simulink model "VCU_CS75_10_9_SteeringTorque"  (R2014a)
settings: Solver=FixedStepDiscrete  StartTime=0.0  StopTime=25  FixedStep=0.0005  RelTol=1e-3
undefined symbols (not defined in the file or in its folder): AutoDrivingReady, ecucoder_acal, I_SW01_L, LaterlAngleCommand, LDW, RemoteAcclPosition
libraries: simulink x880, ec5744lib x37
(part 14 of 30)

== system VCU_CS75_10_9_SteeringTorque/长安CS75底盘程序，20ms一次/Output/CAN0_Tx/to6001/A/Wheel_Speed_RR_Data ==
  Wheel_Speed_RR_Data : Inport
  Constant{1..6} (6 alike) : Constant  Value=0  OutDataTypeStr=uint8
  Wheel_Speed_RR_DataABS : Abs
  Wheel_Speed_RR_DataBitCov : DataTypeConversion  OutDataTypeStr=uint8
  Wheel_Speed_RR_DataCOV : DataTypeConversion  OutDataTypeStr=uint8
  Wheel_Speed_RR_DataCS : ArithShift  BitShiftNumber=-16
  Wheel_Speed_RR_DataConS : Constant  OutDataTypeStr=single
  Wheel_Speed_RR_DataCosR : Constant  Value=0  OutDataTypeStr=uint8
  Wheel_Speed_RR_DataROP : RelationalOperator  Operator=<  OutDataTypeStr=boolean
  Wheel_Speed_RR_DataRon : Rounding  Operator=round
  Wheel_Speed_RR_DataSW : Switch  Criteria=u2 ~= 0
  Wheel_Speed_RR_Data_1sat : Saturate  UpperLimit=65535  LowerLimit=0
  Wheel_Speed_RR_Data_And : simulink/Logic and Bit Operations/Bitwise Operator  logicop=AND  UseBitMask=off  NumInputPorts=2  BitMask=bin2dec('11011001')  BitMaskRealWorld=Stored Integer
  Wheel_Speed_RR_Data_And_C : Constant  Value=255  OutDataTypeStr=uint32
  Wheel_Speed_RR_Data_Convert : DataTypeConversion  OutDataTypeStr=uint32
  Wheel_Speed_RR_Data_D : Product  Inputs=*/
  Wheel_Speed_RR_Data_D1 : Product  Inputs=*/
  Wheel_Speed_RR_Data_F : Constant  Value=0.05625  OutDataTypeStr=single
  Wheel_Speed_RR_Data_L : simulink/Logic and Bit Operations/Bitwise Operator  logicop=AND  UseBitMask=on  BitMask=65535  BitMaskRealWorld=Stored Integer
  Wheel_Speed_RR_Data_O : Constant  Value=0  OutDataTypeStr=single
  Wheel_Speed_RR_Data_S : ArithShift
  Wheel_Speed_RR_Data_sat : Saturate  UpperLimit=200  LowerLimit=-200
  Wheel_Speed_RR_Data_st : Sum  Inputs=+-
  Wheel_Speed_RR_Dataoutput7_C : Constant  Value=256
  Wheel_Speed_RR_Datasubcon : Sum  Inputs=+-
  output1 : Outport
  output2 : Outport  Port=2
  output3 : Outport  Port=3
  output4 : Outport  Port=4
  output5 : Outport  Port=5
  output6 : Outport  Port=6
  output7 : Outport  Port=7
  output8 : Outport  Port=8
  wires:
  Constant6/1 -> output6/1
  Constant5/1 -> output5/1
  Constant4/1 -> output4/1
  Constant3/1 -> output3/1
  Constant2/1 -> output2/1
  Constant1/1 -> output1/1
  Wheel_Speed_RR_DataBitCov/1 -> output8/1
  Wheel_Speed_RR_Data_And/1 -> Wheel_Speed_RR_DataBitCov/1
  Wheel_Speed_RR_Data_And_C/1 -> Wheel_Speed_RR_Data_And/2
  Wheel_Speed_RR_DataCOV/1 -> output7/1
  Wheel_Speed_RR_Data_D1/1 -> Wheel_Speed_RR_DataCOV/1
  Wheel_Speed_RR_Dataoutput7_C/1 -> Wheel_Speed_RR_Data_D1/2
  Wheel_Speed_RR_Data_L/1 -> Wheel_Speed_RR_Data_And/1, Wheel_Speed_RR_Data_D1/1
  Wheel_Speed_RR_Data_Convert/1 -> Wheel_Speed_RR_Data_L/1
  Wheel_Speed_RR_Data_1sat/1 -> Wheel_Speed_RR_Data_Convert/1
  Wheel_Speed_RR_Data_S/1 -> Wheel_Speed_RR_Data_1sat/1
  Wheel_Speed_RR_DataSW/1 -> Wheel_Speed_RR_Data_S/1
  Wheel_Speed_RR_DataROP/1 -> Wheel_Speed_RR_DataSW/2
  Wheel_Speed_RR_Datasubcon/1 -> Wheel_Speed_RR_DataSW/1
  Wheel_Speed_RR_DataABS/1 -> Wheel_Speed_RR_Datasubcon/2
  Wheel_Speed_RR_DataCS/1 -> Wheel_Speed_RR_Datasubcon/1
  Wheel_Speed_RR_DataConS/1 -> Wheel_Speed_RR_DataCS/1
  Wheel_Speed_RR_DataCosR/1 -> Wheel_Speed_RR_DataROP/2
  Wheel_Speed_RR_DataRon/1 -> Wheel_Speed_RR_DataSW/3, Wheel_Speed_RR_DataABS/1, Wheel_Speed_RR_DataROP/1
  Wheel_Speed_RR_Data_D/1 -> Wheel_Speed_RR_DataRon/1
  Wheel_Speed_RR_Data_F/1 -> Wheel_Speed_RR_Data_D/2
  Wheel_Speed_RR_Data_st/1 -> Wheel_Speed_RR_Data_D/1
  Wheel_Speed_RR_Data_O/1 -> Wheel_Speed_RR_Data_st/2
  Wheel_Speed_RR_Data_sat/1 -> Wheel_Speed_RR_Data_st/1
  Wheel_Speed_RR_Data/1 -> Wheel_Speed_RR_Data_sat/1

== system VCU_CS75_10_9_SteeringTorque/长安CS75底盘程序，20ms一次/Output/CAN0_Tx/to6002/B/BrakePeadlState ==
  BrakePeadlState : Inport
  BrakePeadlStateRon : Rounding  Operator=round
  BrakePeadlState_1sat : Saturate  UpperLimit=255  LowerLimit=0
  BrakePeadlState_Convert : DataTypeConversion  OutDataTypeStr=uint8
  BrakePeadlState_Convert1 : DataTypeConversion  OutDataTypeStr=uint32
  BrakePeadlState_D : Product  Inputs=*/
  BrakePeadlState_F : Constant  OutDataTypeStr=single
  BrakePeadlState_L : simulink/Logic and Bit Operations/Bitwise Operator  logicop=AND  UseBitMask=on  BitMask=255  BitMaskRealWorld=Stored Integer
  BrakePeadlState_O : Constant  Value=0  OutDataTypeStr=single
  BrakePeadlState_S : ArithShift
  BrakePeadlState_sat : Saturate  UpperLimit=3  LowerLimit=0
  BrakePeadlState_st : Sum  Inputs=+-
  Constant{1..5,7..8} (7 alike) : Constant  Value=0  OutDataTypeStr=uint8
  output1 : Outport
  output2 : Outport  Port=2
  output3 : Outport  Port=3
  output4 : Outport  Port=4
  output5 : Outport  Port=5
  output6 : Outport  Port=6
  output7 : Outport  Port=7
  output8 : Outport  Port=8
  wires:
  BrakePeadlState/1 -> BrakePeadlState_sat/1
  BrakePeadlState_sat/1 -> BrakePeadlState_st/1
  BrakePeadlState_O/1 -> BrakePeadlState_st/2
  BrakePeadlState_st/1 -> BrakePeadlState_D/1
  BrakePeadlState_F/1 -> BrakePeadlState_D/2
  BrakePeadlState_D/1 -> BrakePeadlStateRon/1
  BrakePeadlStateRon/1 -> BrakePeadlState_S/1
  BrakePeadlState_S/1 -> BrakePeadlState_1sat/1
  BrakePeadlState_1sat/1 -> BrakePeadlState_Convert1/1
  BrakePeadlState_Convert1/1 -> BrakePeadlState_L/1
  BrakePeadlState_L/1 -> BrakePeadlState_Convert/1
  BrakePeadlState_Convert/1 -> output6/1
  Constant1/1 -> output1/1
  Constant2/1 -> output2/1
  Constant3/1 -> output3/1
  Constant4/1 -> output4/1
  Constant5/1 -> output5/1
  Constant7/1 -> output7/1
  Constant8/1 -> output8/1

== system VCU_CS75_10_9_SteeringTorque/长安CS75底盘程序，20ms一次/Output/CAN0_Tx/to6002/B/RemoteDecelerationRequest ==
  RemoteDecelerationRequest : Inport
  Constant{1..7} (7 alike) : Constant  Value=0  OutDataTypeStr=uint8
  RemoteDecelerationRequestRon : Rounding  Operator=round
  RemoteDecelerationRequest_1sat : Saturate  UpperLimit=255  LowerLimit=0
  RemoteDecelerationRequest_Convert : DataTypeConversion  OutDataTypeStr=uint8
  RemoteDecelerationRequest_Convert1 : DataTypeConversion  OutDataTypeStr=uint32
  RemoteDecelerationRequest_D : Product  Inputs=*/
  RemoteDecelerationRequest_F : Constant  Value=0.05  OutDataTypeStr=single
  RemoteDecelerationRequest_L : simulink/Logic and Bit Operations/Bitwise Operator  logicop=AND  UseBitMask=on  BitMask=255  BitMaskRealWorld=Stored Integer
  RemoteDecelerationRequest_O : Constant  Value=0  OutDataTypeStr=single
  RemoteDecelerationRequest_S : ArithShift
  RemoteDecelerationRequest_sat : Saturate  UpperLimit=12.75  LowerLimit=0
  RemoteDecelerationRequest_st : Sum  Inputs=+-
  output1 : Outport
  output2 : Outport  Port=2
  output3 : Outport  Port=3
  output4 : Outport  Port=4
  output5 : Outport  Port=5
  output6 : Outport  Port=6
  output7 : Outport  Port=7
  output8 : Outport  Port=8
  wires:
  RemoteDecelerationRequest/1 -> RemoteDecelerationRequest_sat/1
  RemoteDecelerationRequest_sat/1 -> RemoteDecelerationRequest_st/1
  RemoteDecelerationRequest_O/1 -> RemoteDecelerationRequest_st/2
  RemoteDecelerationRequest_st/1 -> RemoteDecelerationRequest_D/1
  RemoteDecelerationRequest_F/1 -> RemoteDecelerationRequest_D/2
  RemoteDecelerationRequest_D/1 -> RemoteDecelerationRequestRon/1
  RemoteDecelerationRequestRon/1 -> RemoteDecelerationRequest_S/1
  RemoteDecelerationRequest_S/1 -> RemoteDecelerationRequest_1sat/1
  RemoteDecelerationRequest_1sat/1 -> RemoteDecelerationRequest_Convert1/1
  RemoteDecelerationRequest_Convert1/1 -> RemoteDecelerationRequest_L/1
  RemoteDecelerationRequest_L/1 -> RemoteDecelerationRequest_Convert/1
  RemoteDecelerationRequest_Convert/1 -> output8/1
  Constant1/1 -> output1/1
  Constant2/1 -> output2/1
  Constant3/1 -> output3/1
  Constant4/1 -> output4/1
  Constant5/1 -> output5/1
  Constant6/1 -> output6/1
  Constant7/1 -> output7/1

== system VCU_CS75_10_9_SteeringTorque/长安CS75底盘程序，20ms一次/Output/CAN0_Tx/to6002/B/RemoteThrottlePercentage ==
  RemoteThrottlePercentage : Inport
  Constant{1..6,8} (7 alike) : Constant  Value=0  OutDataTypeStr=uint8
  RemoteThrottlePercentageRon : Rounding  Operator=round
  RemoteThrottlePercentage_1sat : Saturate  UpperLimit=255  LowerLimit=0
  RemoteThrottlePercentage_Convert : DataTypeConversion  OutDataTypeStr=uint8
  RemoteThrottlePercentage_Convert1 : DataTypeConversion  OutDataTypeStr=uint32
  RemoteThrottlePercentage_D : Product  Inputs=*/
  RemoteThrottlePercentage_F : Constant  Value=0.4  OutDataTypeStr=single
  RemoteThrottlePercentage_L : simulink/Logic and Bit Operations/Bitwise Operator  logicop=AND  UseBitMask=on  BitMask=255  BitMaskRealWorld=Stored Integer
  RemoteThrottlePercentage_O : Constant  Value=0  OutDataTypeStr=single
  RemoteThrottlePercentage_S : ArithShift
  RemoteThrottlePercentage_sat : Saturate  UpperLimit=100  LowerLimit=0
  RemoteThrottlePercentage_st : Sum  Inputs=+-
  output1 : Outport
  output2 : Outport  Port=2
  output3 : Outport  Port=3
  output4 : Outport  Port=4
  output5 : Outport  Port=5
  output6 : Outport  Port=6
  output7 : Outport  Port=7
  output8 : Outport  Port=8
  wires:
  RemoteThrottlePercentage/1 -> RemoteThrottlePercentage_sat/1
  RemoteThrottlePercentage_sat/1 -> RemoteThrottlePercentage_st/1
  RemoteThrottlePercentage_O/1 -> RemoteThrottlePercentage_st/2
  RemoteThrottlePercentage_st/1 -> RemoteThrottlePercentage_D/1
  RemoteThrottlePercentage_F/1 -> RemoteThrottlePercentage_D/2
  RemoteThrottlePercentage_D/1 -> RemoteThrottlePercentageRon/1
  RemoteThrottlePercentageRon/1 -> RemoteThrottlePercentage_S/1
  RemoteThrottlePercentage_S/1 -> RemoteThrottlePercentage_1sat/1
  RemoteThrottlePercentage_1sat/1 -> RemoteThrottlePercentage_Convert1/1
  RemoteThrottlePercentage_Convert1/1 -> RemoteThrottlePercentage_L/1
  RemoteThrottlePercentage_L/1 -> RemoteThrottlePercentage_Convert/1
  RemoteThrottlePercentage_Convert/1 -> output7/1
  Constant1/1 -> output1/1
  Constant2/1 -> output2/1
  Constant3/1 -> output3/1
  Constant4/1 -> output4/1
  Constant5/1 -> output5/1
  Constant6/1 -> output6/1
  Constant8/1 -> output8/1

== system VCU_CS75_10_9_SteeringTorque/长安CS75底盘程序，20ms一次/Output/CAN0_Tx/to6002/B/Steering_Angle ==
  Steering_Angle : Inport
  Constant{1..2,5..8} (6 alike) : Constant  Value=0  OutDataTypeStr=uint8
  Steering_AngleABS : Abs
  Steering_AngleBitCov : DataTypeConversion  OutDataTypeStr=uint8
  Steering_AngleCOV : DataTypeConversion  OutDataTypeStr=uint8
  Steering_AngleCS : ArithShift  BitShiftNumber=-16
  Steering_AngleConS : Constant  OutDataTypeStr=single
  Steering_AngleCosR : Constant  Value=0  OutDataTypeStr=uint8
  Steering_AngleROP : RelationalOperator  Operator=<  OutDataTypeStr=boolean
  Steering_AngleRon : Rounding  Operator=round
  Steering_AngleSW : Switch  Criteria=u2 ~= 0
  Steering_Angle_1sat : Saturate  UpperLimit=65535  LowerLimit=0
  Steering_Angle_And : simulink/Logic and Bit Operations/Bitwise Operator  logicop=AND  UseBitMask=off  NumInputPorts=2  BitMask=bin2dec('11011001')  BitMaskRealWorld=Stored Integer
  Steering_Angle_And_C : Constant  Value=255  OutDataTypeStr=uint32
  Steering_Angle_Convert : DataTypeConversion  OutDataTypeStr=uint32
  Steering_Angle_D : Product  Inputs=*/
  Steering_Angle_D1 : Product  Inputs=*/
  Steering_Angle_F : Constant  Value=0.1  OutDataTypeStr=single
  Steering_Angle_L : simulink/Logic and Bit Operations/Bitwise Operator  logicop=AND  UseBitMask=on  BitMask=65535  BitMaskRealWorld=Stored Integer
  Steering_Angle_O : Constant  Value=0  OutDataTypeStr=single
  Steering_Angle_S : ArithShift
  Steering_Angle_sat : Saturate  UpperLimit=780  LowerLimit=-780
  Steering_Angle_st : Sum  Inputs=+-
  Steering_Angleoutput3_C : Constant  Value=256
  Steering_Anglesubcon : Sum  Inputs=+-
  output1 : Outport
  output2 : Outport  Port=2
  output3 : Outport  Port=3
  output4 : Outport  Port=4
  output5 : Outport  Port=5
  output6 : Outport  Port=6
  output7 : Outport  Port=7
  output8 : Outport  Port=8
  wires:
  Steering_Angle/1 -> Steering_Angle_sat/1
  Steering_Angle_sat/1 -> Steering_Angle_st/1
  Steering_Angle_O/1 -> Steering_Angle_st/2
  Steering_Angle_st/1 -> Steering_Angle_D/1
  Steering_Angle_F/1 -> Steering_Angle_D/2
  Steering_Angle_D/1 -> Steering_AngleRon/1
  Steering_AngleRon/1 -> Steering_AngleROP/1, Steering_AngleABS/1, Steering_AngleSW/3
  Steering_AngleCosR/1 -> Steering_AngleROP/2
  Steering_AngleConS/1 -> Steering_AngleCS/1
  Steering_AngleCS/1 -> Steering_Anglesubcon/1
  Steering_AngleABS/1 -> Steering_Anglesubcon/2
  Steering_Anglesubcon/1 -> Steering_AngleSW/1
  Steering_AngleROP/1 -> Steering_AngleSW/2
  Steering_AngleSW/1 -> Steering_Angle_S/1
  Steering_Angle_S/1 -> Steering_Angle_1sat/1
  Steering_Angle_1sat/1 -> Steering_Angle_Convert/1
  Steering_Angle_Convert/1 -> Steering_Angle_L/1
  Steering_Angle_L/1 -> Steering_Angle_D1/1, Steering_Angle_And/1
  Steering_Angleoutput3_C/1 -> Steering_Angle_D1/2
  Steering_Angle_D1/1 -> Steering_AngleCOV/1
  Steering_AngleCOV/1 -> output3/1
  Steering_Angle_And_C/1 -> Steering_Angle_And/2
  Steering_Angle_And/1 -> Steering_AngleBitCov/1
  Steering_AngleBitCov/1 -> output4/1
  Constant1/1 -> output1/1
  Constant2/1 -> output2/1
  Constant5/1 -> output5/1
  Constant6/1 -> output6/1
  Constant7/1 -> output7/1
  Constant8/1 -> output8/1

== system VCU_CS75_10_9_SteeringTorque/长安CS75底盘程序，20ms一次/Output/CAN0_Tx/to6002/B/ThrottlePedalPercentage ==
  ThrottlePedalPercentage : Inport
  Constant{1..4,6..8} (7 alike) : Constant  Value=0  OutDataTypeStr=uint8
  ThrottlePedalPercentageRon : Rounding  Operator=round
  ThrottlePedalPercentage_1sat : Saturate  UpperLimit=255  LowerLimit=0
  ThrottlePedalPercentage_Convert : DataTypeConversion  OutDataTypeStr=uint8
  ThrottlePedalPercentage_Convert1 : DataTypeConversion  OutDataTypeStr=uint32
  ThrottlePedalPercentage_D : Product  Inputs=*/
  ThrottlePedalPercentage_F : Constant  Value=0.4  OutDataTypeStr=single
  ThrottlePedalPercentage_L : simulink/Logic and Bit Operations/Bitwise Operator  logicop=AND  UseBitMask=on  BitMask=255  BitMaskRealWorld=Stored Integer
  ThrottlePedalPercentage_O : Constant  Value=0  OutDataTypeStr=single
  ThrottlePedalPercentage_S : ArithShift
  ThrottlePedalPercentage_sat : Saturate  UpperLimit=100  LowerLimit=0
  ThrottlePedalPercentage_st : Sum  Inputs=+-
  output1 : Outport
  output2 : Outport  Port=2
  output3 : Outport  Port=3
  output4 : Outport  Port=4
  output5 : Outport  Port=5
  output6 : Outport  Port=6
  output7 : Outport  Port=7
  output8 : Outport  Port=8
  wires:
  ThrottlePedalPercentage/1 -> ThrottlePedalPercentage_sat/1
  ThrottlePedalPercentage_sat/1 -> ThrottlePedalPercentage_st/1
  ThrottlePedalPercentage_O/1 -> ThrottlePedalPercentage_st/2
  ThrottlePedalPercentage_st/1 -> ThrottlePedalPercentage_D/1
  ThrottlePedalPercentage_F/1 -> ThrottlePedalPercentage_D/2
  ThrottlePedalPercentage_D/1 -> ThrottlePedalPercentageRon/1
  ThrottlePedalPercentageRon/1 -> ThrottlePedalPercentage_S/1
  ThrottlePedalPercentage_S/1 -> ThrottlePedalPercentage_1sat/1
  ThrottlePedalPercentage_1sat/1 -> ThrottlePedalPercentage_Convert1/1
  ThrottlePedalPercentage_Convert1/1 -> ThrottlePedalPercentage_L/1
  ThrottlePedalPercentage_L/1 -> ThrottlePedalPercentage_Convert/1
  ThrottlePedalPercentage_Convert/1 -> output5/1
  Constant1/1 -> output1/1
  Constant2/1 -> output2/1
  Constant3/1 -> output3/1
  Constant4/1 -> output4/1
  Constant6/1 -> output6/1
  Constant7/1 -> output7/1
  Constant8/1 -> output8/1

== system VCU_CS75_10_9_SteeringTorque/长安CS75底盘程序，20ms一次/Output/CAN0_Tx/to6002/B/VehicleSpeed ==
  VehicleSpeed : Inport
  Constant{3..8} (6 alike) : Constant  Value=0  OutDataTypeStr=uint8
  VehicleSpeedABS : Abs
  VehicleSpeedBitCov : DataTypeConversion  OutDataTypeStr=uint8
  VehicleSpeedCOV : DataTypeConversion  OutDataTypeStr=uint8
  VehicleSpeedCS : ArithShift  BitShiftNumber=-16
  VehicleSpeedConS : Constant  OutDataTypeStr=single
  VehicleSpeedCosR : Constant  Value=0  OutDataTypeStr=uint8
  VehicleSpeedROP : RelationalOperator  Operator=<  OutDataTypeStr=boolean
  VehicleSpeedRon : Rounding  Operator=round
  VehicleSpeedSW : Switch  Criteria=u2 ~= 0
  VehicleSpeed_1sat : Saturate  UpperLimit=65535  LowerLimit=0
  VehicleSpeed_And : simulink/Logic and Bit Operations/Bitwise Operator  logicop=AND  UseBitMask=off  NumInputPorts=2  BitMask=bin2dec('11011001')  BitMaskRealWorld=Stored Integer
  VehicleSpeed_And_C : Constant  Value=255  OutDataTypeStr=uint32
  VehicleSpeed_Convert : DataTypeConversion  OutDataTypeStr=uint32
  VehicleSpeed_D : Product  Inputs=*/
  VehicleSpeed_D1 : Product  Inputs=*/
  VehicleSpeed_F : Constant  Value=0.05625  OutDataTypeStr=single
  VehicleSpeed_L : simulink/Logic and Bit Operations/Bitwise Operator  logicop=AND  UseBitMask=on  BitMask=65535  BitMaskRealWorld=Stored Integer
  VehicleSpeed_O : Constant  Value=0  OutDataTypeStr=single
  VehicleSpeed_S : ArithShift
  VehicleSpeed_sat : Saturate  UpperLimit=200  LowerLimit=-200
  VehicleSpeed_st : Sum  Inputs=+-
  VehicleSpeedoutput1_C : Constant  Value=256
  VehicleSpeedsubcon : Sum  Inputs=+-
  output1 : Outport
  output2 : Outport  Port=2
  output3 : Outport  Port=3
  output4 : Outport  Port=4
  output5 : Outport  Port=5
  output6 : Outport  Port=6
  output7 : Outport  Port=7
  output8 : Outport  Port=8
  wires:
  VehicleSpeed/1 -> VehicleSpeed_sat/1
  VehicleSpeed_sat/1 -> VehicleSpeed_st/1
  VehicleSpeed_O/1 -> VehicleSpeed_st/2
  VehicleSpeed_st/1 -> VehicleSpeed_D/1
  VehicleSpeed_F/1 -> VehicleSpeed_D/2
  VehicleSpeed_D/1 -> VehicleSpeedRon/1
  VehicleSpeedRon/1 -> VehicleSpeedROP/1, VehicleSpeedABS/1, VehicleSpeedSW/3
  VehicleSpeedCosR/1 -> VehicleSpeedROP/2
  VehicleSpeedConS/1 -> VehicleSpeedCS/1
  VehicleSpeedCS/1 -> VehicleSpeedsubcon/1
  VehicleSpeedABS/1 -> VehicleSpeedsubcon/2
  VehicleSpeedsubcon/1 -> VehicleSpeedSW/1
  VehicleSpeedROP/1 -> VehicleSpeedSW/2
  VehicleSpeedSW/1 -> VehicleSpeed_S/1
  VehicleSpeed_S/1 -> VehicleSpeed_1sat/1
  VehicleSpeed_1sat/1 -> VehicleSpeed_Convert/1
  VehicleSpeed_Convert/1 -> VehicleSpeed_L/1
  VehicleSpeed_L/1 -> VehicleSpeed_D1/1, VehicleSpeed_And/1
  VehicleSpeedoutput1_C/1 -> VehicleSpeed_D1/2
  VehicleSpeed_D1/1 -> VehicleSpeedCOV/1
  VehicleSpeedCOV/1 -> output1/1
  VehicleSpeed_And_C/1 -> VehicleSpeed_And/2
  VehicleSpeed_And/1 -> VehicleSpeedBitCov/1
  VehicleSpeedBitCov/1 -> output2/1
  Constant3/1 -> output3/1
  Constant4/1 -> output4/1
  Constant5/1 -> output5/1
  Constant6/1 -> output6/1
  Constant7/1 -> output7/1
  Constant8/1 -> output8/1

== system VCU_CS75_10_9_SteeringTorque/长安CS75底盘程序，20ms一次/Output/CAN0_Tx/to6003/C/LateralAcceleration ==
  LateralAcceleration : Inport
  Constant{1..2,4..8} (7 alike) : Constant  Value=0  OutDataTypeStr=uint8
  LateralAccelerationRon : Rounding  Operator=round
  LateralAcceleration_1sat : Saturate  UpperLimit=255  LowerLimit=0
  LateralAcceleration_Convert : DataTypeConversion  OutDataTypeStr=uint8
  LateralAcceleration_Convert1 : DataTypeConversion  OutDataTypeStr=uint32
  LateralAcceleration_D : Product  Inputs=*/
  LateralAcceleration_F : Constant  Value=0.1  OutDataTypeStr=single
  LateralAcceleration_L : simulink/Logic and Bit Operations/Bitwise Operator  logicop=AND  UseBitMask=on  BitMask=255  BitMaskRealWorld=Stored Integer
  LateralAcceleration_O : Constant  Value=-12.7  OutDataTypeStr=single
  LateralAcceleration_S : ArithShift
  LateralAcceleration_sat : Saturate  UpperLimit=12.8  LowerLimit=-12.7
  LateralAcceleration_st : Sum  Inputs=+-
  output1 : Outport
  output2 : Outport  Port=2
  output3 : Outport  Port=3
  output4 : Outport  Port=4
  output5 : Outport  Port=5
  output6 : Outport  Port=6
  output7 : Outport  Port=7
  output8 : Outport  Port=8
  wires:
  LateralAcceleration/1 -> LateralAcceleration_sat/1
  LateralAcceleration_sat/1 -> LateralAcceleration_st/1
  LateralAcceleration_O/1 -> LateralAcceleration_st/2
  LateralAcceleration_st/1 -> LateralAcceleration_D/1
  LateralAcceleration_F/1 -> LateralAcceleration_D/2
  LateralAcceleration_D/1 -> LateralAccelerationRon/1
  LateralAccelerationRon/1 -> LateralAcceleration_S/1
  LateralAcceleration_S/1 -> LateralAcceleration_1sat/1
  LateralAcceleration_1sat/1 -> LateralAcceleration_Convert1/1
  LateralAcceleration_Convert1/1 -> LateralAcceleration_L/1
  LateralAcceleration_L/1 -> LateralAcceleration_Convert/1
  LateralAcceleration_Convert/1 -> output3/1
  Constant1/1 -> output1/1
  Constant2/1 -> output2/1
  Constant4/1 -> output4/1
  Constant5/1 -> output5/1
  Constant6/1 -> output6/1
  Constant7/1 -> output7/1
  Constant8/1 -> output8/1

== system VCU_CS75_10_9_SteeringTorque/长安CS75底盘程序，20ms一次/Output/CAN0_Tx/to6003/C/LongitudinalAcceleration ==
  LongitudinalAcceleration : Inport
  Constant{1..3,6..8} (6 alike) : Constant  Value=0  OutDataTypeStr=uint8
  LongitudinalAccelerationBitCov : DataTypeConversion  OutDataTypeStr=uint8
  LongitudinalAccelerationCOV : DataTypeConversion  OutDataTypeStr=uint8
  LongitudinalAccelerationRon : Rounding  Operator=round
  LongitudinalAcceleration_1sat : Saturate  UpperLimit=65535  LowerLimit=0
  LongitudinalAcceleration_And : simulink/Logic and Bit Operations/Bitwise Operator  logicop=AND  UseBitMask=off  NumInputPorts=2  BitMask=bin2dec('11011001')  BitMaskRealWorld=Stored Integer
  LongitudinalAcceleration_And_C : Constant  Value=255  OutDataTypeStr=uint32
  LongitudinalAcceleration_Convert : DataTypeConversion  OutDataTypeStr=uint32
  LongitudinalAcceleration_D : Product  Inputs=*/
  LongitudinalAcceleration_D1 : Product  Inputs=*/
  LongitudinalAcceleration_F : Constant  Value=0.00048829  OutDataTypeStr=single
  LongitudinalAcceleration_L : simulink/Logic and Bit Operations/Bitwise Operator  logicop=AND  UseBitMask=on  BitMask=65535  BitMaskRealWorld=Stored Integer
  LongitudinalAcceleration_O : Constant  Value=-16  OutDataTypeStr=single
  LongitudinalAcceleration_S : ArithShift
  LongitudinalAcceleration_sat : Saturate  UpperLimit=16.00008515  LowerLimit=-16
  LongitudinalAcceleration_st : Sum  Inputs=+-
  LongitudinalAccelerationoutput4_C : Constant  Value=256
  output1 : Outport
  output2 : Outport  Port=2
  output3 : Outport  Port=3
  output4 : Outport  Port=4
  output5 : Outport  Port=5
  output6 : Outport  Port=6
  output7 : Outport  Port=7
  output8 : Outport  Port=8
  wires:
  LongitudinalAcceleration/1 -> LongitudinalAcceleration_sat/1
  LongitudinalAcceleration_sat/1 -> LongitudinalAcceleration_st/1
  LongitudinalAcceleration_O/1 -> LongitudinalAcceleration_st/2
  LongitudinalAcceleration_st/1 -> LongitudinalAcceleration_D/1
  LongitudinalAcceleration_F/1 -> LongitudinalAcceleration_D/2
  LongitudinalAcceleration_D/1 -> LongitudinalAccelerationRon/1
  LongitudinalAccelerationRon/1 -> LongitudinalAcceleration_S/1
  LongitudinalAcceleration_S/1 -> LongitudinalAcceleration_1sat/1
  LongitudinalAcceleration_1sat/1 -> LongitudinalAcceleration_Convert/1
  LongitudinalAcceleration_Convert/1 -> LongitudinalAcceleration_L/1
  LongitudinalAcceleration_L/1 -> LongitudinalAcceleration_D1/1, LongitudinalAcceleration_And/1
  LongitudinalAccelerationoutput4_C/1 -> LongitudinalAcceleration_D1/2
  LongitudinalAcceleration_D1/1 -> LongitudinalAccelerationCOV/1
  LongitudinalAccelerationCOV/1 -> output4/1
  LongitudinalAcceleration_And_C/1 -> LongitudinalAcceleration_And/2
  LongitudinalAcceleration_And/1 -> LongitudinalAccelerationBitCov/1
  LongitudinalAccelerationBitCov/1 -> output5/1
  Constant1/1 -> output1/1
  Constant2/1 -> output2/1
  Constant3/1 -> output3/1
  Constant6/1 -> output6/1
  Constant7/1 -> output7/1
  Constant8/1 -> output8/1

== system VCU_CS75_10_9_SteeringTorque/长安CS75底盘程序，20ms一次/Output/CAN0_Tx/to6003/C/YawRate ==
  YawRate : Inport
  Constant{3..8} (6 alike) : Constant  Value=0  OutDataTypeStr=uint8
  YawRateBitCov : DataTypeConversion  OutDataTypeStr=uint8
  YawRateCOV : DataTypeConversion  OutDataTypeStr=uint8
  YawRateRon : Rounding  Operator=round
  YawRate_1sat : Saturate  UpperLimit=65535  LowerLimit=0
  YawRate_And : simulink/Logic and Bit Operations/Bitwise Operator  logicop=AND  UseBitMask=off  NumInputPorts=2  BitMask=bin2dec('11011001')  BitMaskRealWorld=Stored Integer
  YawRate_And_C : Constant  Value=255  OutDataTypeStr=uint32
  YawRate_Convert : DataTypeConversion  OutDataTypeStr=uint32
  YawRate_D : Product  Inputs=*/
  YawRate_D1 : Product  Inputs=*/
  YawRate_F : Constant  Value=0.0024719  OutDataTypeStr=single
  YawRate_L : simulink/Logic and Bit Operations/Bitwise Operator  logicop=AND  UseBitMask=on  BitMask=65535  BitMaskRealWorld=Stored Integer
  YawRate_O : Constant  Value=-81  OutDataTypeStr=single
  YawRate_S : ArithShift
  YawRate_sat : Saturate  UpperLimit=80.9959665  LowerLimit=-81
  YawRate_st : Sum  Inputs=+-
  YawRateoutput1_C : Constant  Value=256
  output1 : Outport
  output2 : Outport  Port=2
  output3 : Outport  Port=3
  output4 : Outport  Port=4
  output5 : Outport  Port=5
  output6 : Outport  Port=6
  output7 : Outport  Port=7
  output8 : Outport  Port=8
  wires:
  YawRate/1 -> YawRate_sat/1
  YawRate_sat/1 -> YawRate_st/1
  YawRate_O/1 -> YawRate_st/2
  YawRate_st/1 -> YawRate_D/1
  YawRate_F/1 -> YawRate_D/2
  YawRate_D/1 -> YawRateRon/1
  YawRateRon/1 -> YawRate_S/1
  YawRate_S/1 -> YawRate_1sat/1
  YawRate_1sat/1 -> YawRate_Convert/1
  YawRate_Convert/1 -> YawRate_L/1
  YawRate_L/1 -> YawRate_D1/1, YawRate_And/1
  YawRateoutput1_C/1 -> YawRate_D1/2
  YawRate_D1/1 -> YawRateCOV/1
  YawRateCOV/1 -> output1/1
  YawRate_And_C/1 -> YawRate_And/2
  YawRate_And/1 -> YawRateBitCov/1
  YawRateBitCov/1 -> output2/1
  Constant3/1 -> output3/1
  Constant4/1 -> output4/1
  Constant5/1 -> output5/1
  Constant6/1 -> output6/1
  Constant7/1 -> output7/1
  Constant8/1 -> output8/1

== system VCU_CS75_10_9_SteeringTorque/长安CS75底盘程序，20ms一次/Output/CAN0_Tx/to6004/D/CommandSteering ==
  CommandSteering : Inport
  CommandSteeringABS : Abs
  CommandSteeringBitCov : DataTypeConversion  OutDataTypeStr=uint8
  CommandSteeringCOV : DataTypeConversion  OutDataTypeStr=uint8
  CommandSteeringCS : ArithShift  BitShiftNumber=-16
  CommandSteeringConS : Constant  OutDataTypeStr=single
  CommandSteeringCosR : Constant  Value=0  OutDataTypeStr=uint8
  CommandSteeringROP : RelationalOperator  Operator=<  OutDataTypeStr=boolean
  CommandSteeringRon : Rounding  Operator=round
  CommandSteeringSW : Switch  Criteria=u2 ~= 0
  CommandSteering_1sat : Saturate  UpperLimit=65535  LowerLimit=0
  CommandSteering_And : simulink/Logic and Bit Operations/Bitwise Operator  logicop=AND  UseBitMask=off  NumInputPorts=2  BitMask=bin2dec('11011001')  BitMaskRealWorld=Stored Integer
  CommandSteering_And_C : Constant  Value=255  OutDataTypeStr=uint32
  CommandSteering_Convert : DataTypeConversion  OutDataTypeStr=uint32
  CommandSteering_D : Product  Inputs=*/
  CommandSteering_D1 : Product  Inputs=*/
  CommandSteering_F : Constant  Value=0.1  OutDataTypeStr=single
  CommandSteering_L : simulink/Logic and Bit Operations/Bitwise Operator  logicop=AND  UseBitMask=on  BitMask=65535  BitMaskRealWorld=Stored Integer
  CommandSteering_O : Constant  Value=0  OutDataTypeStr=single
  CommandSteering_S : ArithShift
  CommandSteering_sat : Saturate  UpperLimit=780  LowerLimit=-780
  CommandSteering_st : Sum  Inputs=+-
  CommandSteeringoutput3_C : Constant  Value=256
  CommandSteeringsubcon : Sum  Inputs=+-
  Constant{1..2,5..8} (6 alike) : Constant  Value=0  OutDataTypeStr=uint8
  output1 : Outport
  output2 : Outport  Port=2
  output3 : Outport  Port=3
  output4 : Outport  Port=4
  output5 : Outport  Port=5
  output6 : Outport  Port=6
  output7 : Outport  Port=7
  output8 : Outport  Port=8
  wires:
  Constant8/1 -> output8/1
  Constant7/1 -> output7/1
  Constant6/1 -> output6/1
  Constant5/1 -> output5/1
  Constant2/1 -> output2/1
  Constant1/1 -> output1/1
  CommandSteeringBitCov/1 -> output4/1
  CommandSteering_And/1 -> CommandSteeringBitCov/1
  CommandSteering_And_C/1 -> CommandSteering_And/2
  CommandSteeringCOV/1 -> output3/1
  CommandSteering_D1/1 -> CommandSteeringCOV/1
  CommandSteeringoutput3_C/1 -> CommandSteering_D1/2
  CommandSteering_L/1 -> CommandSteering_And/1, CommandSteering_D1/1
  CommandSteering_Convert/1 -> CommandSteering_L/1
  CommandSteering_1sat/1 -> CommandSteering_Convert/1
  CommandSteering_S/1 -> CommandSteering_1sat/1
  CommandSteeringSW/1 -> CommandSteering_S/1
  CommandSteeringROP/1 -> CommandSteeringSW/2
  CommandSteeringsubcon/1 -> CommandSteeringSW/1
  CommandSteeringABS/1 -> CommandSteeringsubcon/2
  CommandSteeringCS/1 -> CommandSteeringsubcon/1
  CommandSteeringConS/1 -> CommandSteeringCS/1
  CommandSteeringCosR/1 -> CommandSteeringROP/2
  CommandSteeringRon/1 -> CommandSteeringSW/3, CommandSteeringABS/1, CommandSteeringROP/1
  CommandSteering_D/1 -> CommandSteeringRon/1
  CommandSteering_F/1 -> CommandSteering_D/2
  CommandSteering_st/1 -> CommandSteering_D/1
  CommandSteering_O/1 -> CommandSteering_st/2
  CommandSteering_sat/1 -> CommandSteering_st/1
  CommandSteering/1 -> CommandSteering_sat/1

== system VCU_CS75_10_9_SteeringTorque/长安CS75底盘程序，20ms一次/Output/CAN0_Tx/to6004/D/Command_ACC ==
  Command_ACC : Inport
  Command_ACCABS : Abs
  Command_ACCBitCov : DataTypeConversion  OutDataTypeStr=uint8
  Command_ACCCOV : DataTypeConversion  OutDataTypeStr=uint8
  Command_ACCCS : ArithShift  BitShiftNumber=-16
  Command_ACCConS : Constant  OutDataTypeStr=single
  Command_ACCCosR : Constant  Value=0  OutDataTypeStr=uint8
  Command_ACCROP : RelationalOperator  Operator=<  OutDataTypeStr=boolean
  Command_ACCRon : Rounding  Operator=round
  Command_ACCSW : Switch  Criteria=u2 ~= 0
  Command_ACC_1sat : Saturate  UpperLimit=65535  LowerLimit=0
  Command_ACC_And : simulink/Logic and Bit Operations/Bitwise Operator  logicop=AND  UseBitMask=off  NumInputPorts=2  BitMask=bin2dec('11011001')  BitMaskRealWorld=Stored Integer
  Command_ACC_And_C : Constant  Value=255  OutDataTypeStr=uint32
  Command_ACC_Convert : DataTypeConversion  OutDataTypeStr=uint32
  Command_ACC_D : Product  Inputs=*/
  Command_ACC_D1 : Product  Inputs=*/
  Command_ACC_F : Constant  Value=0.005  OutDataTypeStr=single
  Command_ACC_L : simulink/Logic and Bit Operations/Bitwise Operator  logicop=AND  UseBitMask=on  BitMask=65535  BitMaskRealWorld=Stored Integer
  Command_ACC_O : Constant  Value=0  OutDataTypeStr=single
  Command_ACC_S : ArithShift
  Command_ACC_sat : Saturate  UpperLimit=100  LowerLimit=-10
  Command_ACC_st : Sum  Inputs=+-
  Command_ACCoutput1_C : Constant  Value=256
  Command_ACCsubcon : Sum  Inputs=+-
  Constant{3..8} (6 alike) : Constant  Value=0  OutDataTypeStr=uint8
  output1 : Outport
  output2 : Outport  Port=2
  output3 : Outport  Port=3
  output4 : Outport  Port=4
  output5 : Outport  Port=5
  output6 : Outport  Port=6
  output7 : Outport  Port=7
  output8 : Outport  Port=8
  wires:
  Constant8/1 -> output8/1
  Constant7/1 -> output7/1
  Constant6/1 -> output6/1
  Constant5/1 -> output5/1
  Constant4/1 -> output4/1
  Constant3/1 -> output3/1
  Command_ACCBitCov/1 -> output2/1
  Command_ACC_And/1 -> Command_ACCBitCov/1
  Command_ACC_And_C/1 -> Command_ACC_And/2
  Command_ACCCOV/1 -> output1/1
  Command_ACC_D1/1 -> Command_ACCCOV/1
  Command_ACCoutput1_C/1 -> Command_ACC_D1/2
  Command_ACC_L/1 -> Command_ACC_And/1, Command_ACC_D1/1
  Command_ACC_Convert/1 -> Command_ACC_L/1
  Command_ACC_1sat/1 -> Command_ACC_Convert/1
  Command_ACC_S/1 -> Command_ACC_1sat/1
  Command_ACCSW/1 -> Command_ACC_S/1
  Command_ACCROP/1 -> Command_ACCSW/2
  Command_ACCsubcon/1 -> Command_ACCSW/1
  Command_ACCABS/1 -> Command_ACCsubcon/2
  Command_ACCCS/1 -> Command_ACCsubcon/1
  Command_ACCConS/1 -> Command_ACCCS/1
  Command_ACCCosR/1 -> Command_ACCROP/2
  Command_ACCRon/1 -> Command_ACCSW/3, Command_ACCABS/1, Command_ACCROP/1
  Command_ACC_D/1 -> Command_ACCRon/1
  Command_ACC_F/1 -> Command_ACC_D/2
  Command_ACC_st/1 -> Command_ACC_D/1
  Command_ACC_O/1 -> Command_ACC_st/2
  Command_ACC_sat/1 -> Command_ACC_st/1
  Command_ACC/1 -> Command_ACC_sat/1

== system VCU_CS75_10_9_SteeringTorque/长安CS75底盘程序，20ms一次/Output/CAN0_Tx/to6004/D/ControllerErrorState ==
  ControllerErrorState : Inport
  Constant{1..4,6..8} (7 alike) : Constant  Value=0  OutDataTypeStr=uint8
  ControllerErrorStateRon : Rounding  Operator=round
  ControllerErrorState_1sat : Saturate  UpperLimit=255  LowerLimit=0
  ControllerErrorState_Convert : DataTypeConversion  OutDataTypeStr=uint8
  ControllerErrorState_Convert1 : DataTypeConversion  OutDataTypeStr=uint32
  ControllerErrorState_D : Product  Inputs=*/
  ControllerErrorState_F : Constant  OutDataTypeStr=single
  ControllerErrorState_L : simulink/Logic and Bit Operations/Bitwise Operator  logicop=AND  UseBitMask=on  BitMask=255  BitMaskRealWorld=Stored Integer
  ControllerErrorState_O : Constant  Value=0  OutDataTypeStr=single
  ControllerErrorState_S : ArithShift
  ControllerErrorState_sat : Saturate  UpperLimit=255  LowerLimit=0
  ControllerErrorState_st : Sum  Inputs=+-
  output1 : Outport
  output2 : Outport  Port=2
  output3 : Outport  Port=3
  output4 : Outport  Port=4
  output5 : Outport  Port=5
  output6 : Outport  Port=6
  output7 : Outport  Port=7
  output8 : Outport  Port=8
  wires:
  Constant8/1 -> output8/1
  Constant7/1 -> output7/1
  Constant6/1 -> output6/1
  Constant4/1 -> output4/1
  Constant3/1 -> output3/1
  Constant2/1 -> output2/1
  Constant1/1 -> output1/1
  ControllerErrorState_Convert/1 -> output5/1
  ControllerErrorState_L/1 -> ControllerErrorState_Convert/1
  ControllerErrorState_Convert1/1 -> ControllerErrorState_L/1
  ControllerErrorState_1sat/1 -> ControllerErrorState_Convert1/1
  ControllerErrorState_S/1 -> ControllerErrorState_1sat/1
  ControllerErrorStateRon/1 -> ControllerErrorState_S/1
  ControllerErrorState_D/1 -> ControllerErrorStateRon/1
  ControllerErrorState_F/1 -> ControllerErrorState_D/2
  ControllerErrorState_st/1 -> ControllerErrorState_D/1
  ControllerErrorState_O/1 -> ControllerErrorState_st/2
  ControllerErrorState_sat/1 -> ControllerErrorState_st/1
  ControllerErrorState/1 -> ControllerErrorState_sat/1

== system VCU_CS75_10_9_SteeringTorque/长安CS75底盘程序，20ms一次/Output/CAN0_Tx/to6004/D/FSM_CurrentState ==
  FSM_CurrentState : Inport
  Constant{1..5,7..8} (7 alike) : Constant  Value=0  OutDataTypeStr=uint8
  FSM_CurrentStateRon : Rounding  Operator=round
  FSM_CurrentState_1sat : Saturate  UpperLimit=255  LowerLimit=0
  FSM_CurrentState_Convert : DataTypeConversion  OutDataTypeStr=uint8
  FSM_CurrentState_Convert1 : DataTypeConversion  OutDataTypeStr=uint32
  FSM_CurrentState_D : Product  Inputs=*/
  FSM_CurrentState_F : Constant  OutDataTypeStr=single
  FSM_CurrentState_L : simulink/Logic and Bit Operations/Bitwise Operator  logicop=AND  UseBitMask=on  BitMask=255  BitMaskRealWorld=Stored Integer
  FSM_CurrentState_O : Constant  Value=0  OutDataTypeStr=single
  FSM_CurrentState_S : ArithShift
  FSM_CurrentState_sat : Saturate  UpperLimit=3  LowerLimit=0
  FSM_CurrentState_st : Sum  Inputs=+-
  output1 : Outport
  output2 : Outport  Port=2
  output3 : Outport  Port=3
  output4 : Outport  Port=4
  output5 : Outport  Port=5
  output6 : Outport  Port=6
  output7 : Outport  Port=7
  output8 : Outport  Port=8
  wires:
  Constant8/1 -> output8/1
  Constant7/1 -> output7/1
  Constant5/1 -> output5/1
  Constant4/1 -> output4/1
  Constant3/1 -> output3/1
  Constant2/1 -> output2/1
  Constant1/1 -> output1/1
  FSM_CurrentState_Convert/1 -> output6/1
  FSM_CurrentState_L/1 -> FSM_CurrentState_Convert/1
  FSM_CurrentState_Convert1/1 -> FSM_CurrentState_L/1
  FSM_CurrentState_1sat/1 -> FSM_CurrentState_Convert1/1
  FSM_CurrentState_S/1 -> FSM_CurrentState_1sat/1
  FSM_CurrentStateRon/1 -> FSM_CurrentState_S/1
  FSM_CurrentState_D/1 -> FSM_CurrentStateRon/1
  FSM_CurrentState_F/1 -> FSM_CurrentState_D/2
  FSM_CurrentState_st/1 -> FSM_CurrentState_D/1
  FSM_CurrentState_O/1 -> FSM_CurrentState_st/2
  FSM_CurrentState_sat/1 -> FSM_CurrentState_st/1
  FSM_CurrentState/1 -> FSM_CurrentState_sat/1

== system VCU_CS75_10_9_SteeringTorque/长安CS75底盘程序，20ms一次/Output/CAN0_Tx/to6004/D/LateralAutoDrivingSwitch ==
  LateralAutoDrivingSwitch : Inport
  Constant{1..6,8} (7 alike) : Constant  Value=0  OutDataTypeStr=uint8
  LateralAutoDrivingSwitchRon : Rounding  Operator=round
  LateralAutoDrivingSwitch_1sat : Saturate  UpperLimit=255  LowerLimit=0
  LateralAutoDrivingSwitch_Convert : DataTypeConversion  OutDataTypeStr=uint8
  LateralAutoDrivingSwitch_Convert1 : DataTypeConversion  OutDataTypeStr=uint32
  LateralAutoDrivingSwitch_D : Product  Inputs=*/
  LateralAutoDrivingSwitch_F : Constant  OutDataTypeStr=single
  LateralAutoDrivingSwitch_L : simulink/Logic and Bit Operations/Bitwise Operator  logicop=AND  UseBitMask=on  BitMask=255  BitMaskRealWorld=Stored Integer
  LateralAutoDrivingSwitch_O : Constant  Value=0  OutDataTypeStr=single
  LateralAutoDrivingSwitch_S : ArithShift
  LateralAutoDrivingSwitch_sat : Saturate  UpperLimit=1  LowerLimit=0
  LateralAutoDrivingSwitch_st : Sum  Inputs=+-
  output1 : Outport
  output2 : Outport  Port=2
  output3 : Outport  Port=3
  output4 : Outport  Port=4
  output5 : Outport  Port=5
  output6 : Outport  Port=6
  output7 : Outport  Port=7
  output8 : Outport  Port=8
  wires:
  Constant8/1 -> output8/1
  Constant6/1 -> output6/1
  Constant5/1 -> output5/1
  Constant4/1 -> output4/1
  Constant3/1 -> output3/1
  Constant2/1 -> output2/1
  Constant1/1 -> output1/1
  LateralAutoDrivingSwitch_Convert/1 -> output7/1
  LateralAutoDrivingSwitch_L/1 -> LateralAutoDrivingSwitch_Convert/1
  LateralAutoDrivingSwitch_Convert1/1 -> LateralAutoDrivingSwitch_L/1
  LateralAutoDrivingSwitch_1sat/1 -> LateralAutoDrivingSwitch_Convert1/1
  LateralAutoDrivingSwitch_S/1 -> LateralAutoDrivingSwitch_1sat/1
  LateralAutoDrivingSwitchRon/1 -> LateralAutoDrivingSwitch_S/1
  LateralAutoDrivingSwitch_D/1 -> LateralAutoDrivingSwitchRon/1
  LateralAutoDrivingSwitch_F/1 -> LateralAutoDrivingSwitch_D/2
  LateralAutoDrivingSwitch_st/1 -> LateralAutoDrivingSwitch_D/1
  LateralAutoDrivingSwitch_O/1 -> LateralAutoDrivingSwitch_st/2
  LateralAutoDrivingSwitch_sat/1 -> LateralAutoDrivingSwitch_st/1
  LateralAutoDrivingSwitch/1 -> LateralAutoDrivingSwitch_sat/1

== system VCU_CS75_10_9_SteeringTorque/长安CS75底盘程序，20ms一次/Output/CAN0_Tx/to6004/D/LongitudinalAutoDrivingState ==
  LongitudinalAutoDrivingState : Inport
  Constant{1..7} (7 alike) : Constant  Value=0  OutDataTypeStr=uint8
  LongitudinalAutoDrivingStateRon : Rounding  Operator=round
  LongitudinalAutoDrivingState_1sat : Saturate  UpperLimit=255  LowerLimit=0
  LongitudinalAutoDrivingState_Convert : DataTypeConversion  OutDataTypeStr=uint8
  LongitudinalAutoDrivingState_Convert1 : DataTypeConversion  OutDataTypeStr=uint32
  LongitudinalAutoDrivingState_D : Product  Inputs=*/
  LongitudinalAutoDrivingState_F : Constant  OutDataTypeStr=single
  LongitudinalAutoDrivingState_L : simulink/Logic and Bit Operations/Bitwise Operator  logicop=AND  UseBitMask=on  BitMask=255  BitMaskRealWorld=Stored Integer
  LongitudinalAutoDrivingState_O : Constant  Value=0  OutDataTypeStr=single
  LongitudinalAutoDrivingState_S : ArithShift
  LongitudinalAutoDrivingState_sat : Saturate  UpperLimit=1  LowerLimit=0
  LongitudinalAutoDrivingState_st : Sum  Inputs=+-
  output1 : Outport
  output2 : Outport  Port=2
  output3 : Outport  Port=3
  output4 : Outport  Port=4
  output5 : Outport  Port=5
  output6 : Outport  Port=6
  output7 : Outport  Port=7
  output8 : Outport  Port=8
  wires:
  Constant7/1 -> output7/1
  Constant6/1 -> output6/1
  Constant5/1 -> output5/1
  Constant4/1 -> output4/1
  Constant3/1 -> output3/1
  Constant2/1 -> output2/1
  Constant1/1 -> output1/1
  LongitudinalAutoDrivingState_Convert/1 -> output8/1
  LongitudinalAutoDrivingState_L/1 -> LongitudinalAutoDrivingState_Convert/1
  LongitudinalAutoDrivingState_Convert1/1 -> LongitudinalAutoDrivingState_L/1
  LongitudinalAutoDrivingState_1sat/1 -> LongitudinalAutoDrivingState_Convert1/1
  LongitudinalAutoDrivingState_S/1 -> LongitudinalAutoDrivingState_1sat/1
  LongitudinalAutoDrivingStateRon/1 -> LongitudinalAutoDrivingState_S/1
  LongitudinalAutoDrivingState_D/1 -> LongitudinalAutoDrivingStateRon/1
  LongitudinalAutoDrivingState_F/1 -> LongitudinalAutoDrivingState_D/2
  LongitudinalAutoDrivingState_st/1 -> LongitudinalAutoDrivingState_D/1
  LongitudinalAutoDrivingState_O/1 -> LongitudinalAutoDrivingState_st/2
  LongitudinalAutoDrivingState_sat/1 -> LongitudinalAutoDrivingState_st/1
  LongitudinalAutoDrivingState/1 -> LongitudinalAutoDrivingState_sat/1

== system VCU_CS75_10_9_SteeringTorque/长安CS75底盘程序，20ms一次/Output/CAN1_Tx/to28D/LAS_28D/CRC ==
  CRC : Inport
  CRCRon : Rounding  Operator=round
  CRC_1sat : Saturate  UpperLimit=255  LowerLimit=0
  CRC_Convert : DataTypeConversion  OutDataTypeStr=uint8
  CRC_Convert1 : DataTypeConversion  OutDataTypeStr=uint32
  CRC_D : Product  Inputs=*/
  CRC_F : Constant  OutDataTypeStr=single
  CRC_L : simulink/Logic and Bit Operations/Bitwise Operator  logicop=AND  UseBitMask=on  BitMask=255  BitMaskRealWorld=Stored Integer
  CRC_O : Constant  Value=0  OutDataTypeStr=single
  CRC_S : ArithShift
  CRC_sat : Saturate  UpperLimit=0  LowerLimit=0
  CRC_st : Sum  Inputs=+-
  Constant{1..7} (7 alike) : Constant  Value=0  OutDataTypeStr=uint8
  output1 : Outport
  output2 : Outport  Port=2
  output3 : Outport  Port=3
  output4 : Outport  Port=4
  output5 : Outport  Port=5
  output6 : Outport  Port=6
  output7 : Outport  Port=7
  output8 : Outport  Port=8
  wires:
  CRC/1 -> CRC_sat/1
  CRC_sat/1 -> CRC_st/1
  CRC_O/1 -> CRC_st/2
  CRC_st/1 -> CRC_D/1
  CRC_F/1 -> CRC_D/2
  CRC_D/1 -> CRCRon/1
  CRCRon/1 -> CRC_S/1
  CRC_S/1 -> CRC_1sat/1
  CRC_1sat/1 -> CRC_Convert1/1
  CRC_Convert1/1 -> CRC_L/1
  CRC_L/1 -> CRC_Convert/1
  CRC_Convert/1 -> output8/1
  Constant1/1 -> output1/1
  Constant2/1 -> output2/1
  Constant3/1 -> output3/1
  Constant4/1 -> output4/1
  Constant5/1 -> output5/1
  Constant6/1 -> output6/1
  Constant7/1 -> output7/1

== system VCU_CS75_10_9_SteeringTorque/长安CS75底盘程序，20ms一次/Output/CAN1_Tx/to28D/LAS_28D/LAS_CaliStatus ==
  LAS_CaliStatus : Inport
  Constant{1,3..8} (7 alike) : Constant  Value=0  OutDataTypeStr=uint8
  LAS_CaliStatusRon : Rounding  Operator=round
  LAS_CaliStatus_1sat : Saturate  UpperLimit=3  LowerLimit=0
  LAS_CaliStatus_Convert : DataTypeConversion  OutDataTypeStr=uint8
  LAS_CaliStatus_Convert1 : DataTypeConversion  OutDataTypeStr=uint32
  LAS_CaliStatus_D : Product  Inputs=*/
  LAS_CaliStatus_F : Constant  OutDataTypeStr=single
  LAS_CaliStatus_L : simulink/Logic and Bit Operations/Bitwise Operator  logicop=AND  UseBitMask=on  BitMask=3  BitMaskRealWorld=Stored Integer
  LAS_CaliStatus_O : Constant  Value=0  OutDataTypeStr=single
  LAS_CaliStatus_S : ArithShift
  LAS_CaliStatus_sat : Saturate  UpperLimit=0  LowerLimit=0
  LAS_CaliStatus_st : Sum  Inputs=+-
  output1 : Outport
  output2 : Outport  Port=2
  output3 : Outport  Port=3
  output4 : Outport  Port=4
  output5 : Outport  Port=5
  output6 : Outport  Port=6
  output7 : Outport  Port=7
  output8 : Outport  Port=8
  wires:
  LAS_CaliStatus/1 -> LAS_CaliStatus_sat/1
  LAS_CaliStatus_sat/1 -> LAS_CaliStatus_st/1
  LAS_CaliStatus_O/1 -> LAS_CaliStatus_st/2
  LAS_CaliStatus_st/1 -> LAS_CaliStatus_D/1
  LAS_CaliStatus_F/1 -> LAS_CaliStatus_D/2
  LAS_CaliStatus_D/1 -> LAS_CaliStatusRon/1
  LAS_CaliStatusRon/1 -> LAS_CaliStatus_S/1
  LAS_CaliStatus_S/1 -> LAS_CaliStatus_1sat/1
  LAS_CaliStatus_1sat/1 -> LAS_CaliStatus_Convert1/1
  LAS_CaliStatus_Convert1/1 -> LAS_CaliStatus_L/1
  LAS_CaliStatus_L/1 -> LAS_CaliStatus_Convert/1
  LAS_CaliStatus_Convert/1 -> output2/1
  Constant1/1 -> output1/1
  Constant3/1 -> output3/1
  Constant4/1 -> output4/1
  Constant5/1 -> output5/1
  Constant6/1 -> output6/1
  Constant7/1 -> output7/1
  Constant8/1 -> output8/1

== system VCU_CS75_10_9_SteeringTorque/长安CS75底盘程序，20ms一次/Output/CAN1_Tx/to28D/LAS_28D/LAS_DFDFailed ==
  LAS_DFDFailed : Inport
  Constant{1,3..8} (7 alike) : Constant  Value=0  OutDataTypeStr=uint8
  LAS_DFDFailedRon : Rounding  Operator=round
  LAS_DFDFailed_1sat : Saturate  UpperLimit=8  LowerLimit=0
  LAS_DFDFailed_Convert : DataTypeConversion  OutDataTypeStr=uint8
  LAS_DFDFailed_Convert1 : DataTypeConversion  OutDataTypeStr=uint32
  LAS_DFDFailed_D : Product  Inputs=*/
  LAS_DFDFailed_F : Constant  OutDataTypeStr=single
  LAS_DFDFailed_L : simulink/Logic and Bit Operations/Bitwise Operator  logicop=AND  UseBitMask=on  BitMask=8  BitMaskRealWorld=Stored Integer
  LAS_DFDFailed_O : Constant  Value=0  OutDataTypeStr=single
  LAS_DFDFailed_S : ArithShift  BitShiftNumber=-3
  LAS_DFDFailed_sat : Saturate  UpperLimit=0  LowerLimit=0
  LAS_DFDFailed_st : Sum  Inputs=+-
  output1 : Outport
  output2 : Outport  Port=2
  output3 : Outport  Port=3
  output4 : Outport  Port=4
  output5 : Outport  Port=5
  output6 : Outport  Port=6
  output7 : Outport  Port=7
  output8 : Outport  Port=8
  wires:
  LAS_DFDFailed/1 -> LAS_DFDFailed_sat/1
  LAS_DFDFailed_sat/1 -> LAS_DFDFailed_st/1
  LAS_DFDFailed_O/1 -> LAS_DFDFailed_st/2
  LAS_DFDFailed_st/1 -> LAS_DFDFailed_D/1
  LAS_DFDFailed_F/1 -> LAS_DFDFailed_D/2
  LAS_DFDFailed_D/1 -> LAS_DFDFailedRon/1
  LAS_DFDFailedRon/1 -> LAS_DFDFailed_S/1
  LAS_DFDFailed_S/1 -> LAS_DFDFailed_1sat/1
  LAS_DFDFailed_1sat/1 -> LAS_DFDFailed_Convert1/1
  LAS_DFDFailed_Convert1/1 -> LAS_DFDFailed_L/1
  LAS_DFDFailed_L/1 -> LAS_DFDFailed_Convert/1
  LAS_DFDFailed_Convert/1 -> output2/1
  Constant1/1 -> output1/1
  Constant3/1 -> output3/1
  Constant4/1 -> output4/1
  Constant5/1 -> output5/1
  Constant6/1 -> output6/1
  Constant7/1 -> output7/1
  Constant8/1 -> output8/1

== system VCU_CS75_10_9_SteeringTorque/长安CS75底盘程序，20ms一次/Output/CAN1_Tx/to28D/LAS_28D/LAS_DFDWarning ==
  LAS_DFDWarning : Inport
  Constant{1..3,5..8} (7 alike) : Constant  Value=0  OutDataTypeStr=uint8
  LAS_DFDWarningRon : Rounding  Operator=round
  LAS_DFDWarning_1sat : Saturate  UpperLimit=3  LowerLimit=0
  LAS_DFDWarning_Convert : DataTypeConversion  OutDataTypeStr=uint8
  LAS_DFDWarning_Convert1 : DataTypeConversion  OutDataTypeStr=uint32
  LAS_DFDWarning_D : Product  Inputs=*/
  LAS_DFDWarning_F : Constant  OutDataTypeStr=single
  LAS_DFDWarning_L : simulink/Logic and Bit Operations/Bitwise Operator  logicop=AND  UseBitMask=on  BitMask=3  BitMaskRealWorld=Stored Integer
  LAS_DFDWarning_O : Constant  Value=0  OutDataTypeStr=single
  LAS_DFDWarning_S : ArithShift
  LAS_DFDWarning_sat : Saturate  UpperLimit=0  LowerLimit=0
  LAS_DFDWarning_st : Sum  Inputs=+-
  output1 : Outport
  output2 : Outport  Port=2
  output3 : Outport  Port=3
  output4 : Outport  Port=4
  output5 : Outport  Port=5
  output6 : Outport  Port=6
  output7 : Outport  Port=7
  output8 : Outport  Port=8
  wires:
  LAS_DFDWarning/1 -> LAS_DFDWarning_sat/1
  LAS_DFDWarning_sat/1 -> LAS_DFDWarning_st/1
  LAS_DFDWarning_O/1 -> LAS_DFDWarning_st/2
  LAS_DFDWarning_st/1 -> LAS_DFDWarning_D/1
  LAS_DFDWarning_F/1 -> LAS_DFDWarning_D/2
  LAS_DFDWarning_D/1 -> LAS_DFDWarningRon/1
  LAS_DFDWarningRon/1 -> LAS_DFDWarning_S/1
  LAS_DFDWarning_S/1 -> LAS_DFDWarning_1sat/1
  LAS_DFDWarning_1sat/1 -> LAS_DFDWarning_Convert1/1
  LAS_DFDWarning_Convert1/1 -> LAS_DFDWarning_L/1
  LAS_DFDWarning_L/1 -> LAS_DFDWarning_Convert/1
  LAS_DFDWarning_Convert/1 -> output4/1
  Constant1/1 -> output1/1
  Constant2/1 -> output2/1
  Constant3/1 -> output3/1
  Constant5/1 -> output5/1
  Constant6/1 -> output6/1
  Constant7/1 -> output7/1
  Constant8/1 -> output8/1

== system VCU_CS75_10_9_SteeringTorque/长安CS75底盘程序，20ms一次/Output/CAN1_Tx/to28D/LAS_28D/LAS_LASFailed ==
  LAS_LASFailed : Inport
  Constant{1..3,5..8} (7 alike) : Constant  Value=0  OutDataTypeStr=uint8
  LAS_LASFailedRon : Rounding  Operator=round
  LAS_LASFailed_1sat : Saturate  UpperLimit=12  LowerLimit=0
  LAS_LASFailed_Convert : DataTypeConversion  OutDataTypeStr=uint8
  LAS_LASFailed_Convert1 : DataTypeConversion  OutDataTypeStr=uint32
  LAS_LASFailed_D : Product  Inputs=*/
  LAS_LASFailed_F : Constant  OutDataTypeStr=single
  LAS_LASFailed_L : simulink/Logic and Bit Operations/Bitwise Operator  logicop=AND  UseBitMask=on  BitMask=12  BitMaskRealWorld=Stored Integer
  LAS_LASFailed_O : Constant  Value=0  OutDataTypeStr=single
  LAS_LASFailed_S : ArithShift  BitShiftNumber=-2
  LAS_LASFailed_sat : Saturate  UpperLimit=0  LowerLimit=0
  LAS_LASFailed_st : Sum  Inputs=+-
  output1 : Outport
  output2 : Outport  Port=2
  output3 : Outport  Port=3
  output4 : Outport  Port=4
  output5 : Outport  Port=5
  output6 : Outport  Port=6
  output7 : Outport  Port=7
  output8 : Outport  Port=8
  wires:
  LAS_LASFailed/1 -> LAS_LASFailed_sat/1
  LAS_LASFailed_sat/1 -> LAS_LASFailed_st/1
  LAS_LASFailed_O/1 -> LAS_LASFailed_st/2
  LAS_LASFailed_st/1 -> LAS_LASFailed_D/1
  LAS_LASFailed_F/1 -> LAS_LASFailed_D/2
  LAS_LASFailed_D/1 -> LAS_LASFailedRon/1
  LAS_LASFailedRon/1 -> LAS_LASFailed_S/1
  LAS_LASFailed_S/1 -> LAS_LASFailed_1sat/1
  LAS_LASFailed_1sat/1 -> LAS_LASFailed_Convert1/1
  LAS_LASFailed_Convert1/1 -> LAS_LASFailed_L/1
  LAS_LASFailed_L/1 -> LAS_LASFailed_Convert/1
  LAS_LASFailed_Convert/1 -> output4/1
  Constant1/1 -> output1/1
  Constant2/1 -> output2/1
  Constant3/1 -> output3/1
  Constant5/1 -> output5/1
  Constant6/1 -> output6/1
  Constant7/1 -> output7/1
  Constant8/1 -> output8/1
